simulink model "polaczenie"  (R2013a)
settings: Solver=FixedStepDiscrete  StartTime=0.0  StopTime=inf  FixedStep=0.01  RelTol=1e-3
InitFcn:
  | InitFcn
StopFcn:
  | StopFcn
libraries: aerolibtransform2 x2, aerolibobsolete x2, aerolibconvert2 x2, instrumentlib x2, dspmtrx3 x2
settings Model: Creator=Antonio  LastModifiedBy=Antonio
settings SolverCC: AutoInsertRateTranBlk=on  InsertRTBMode=Always
settings OptimizationCC: LocalBlockOutputs=off  SimCompilerOptimization=On
settings SFSimCC: SFSimEnableDebug=off
settings RTWCC: RTWCompilerOptimization=On

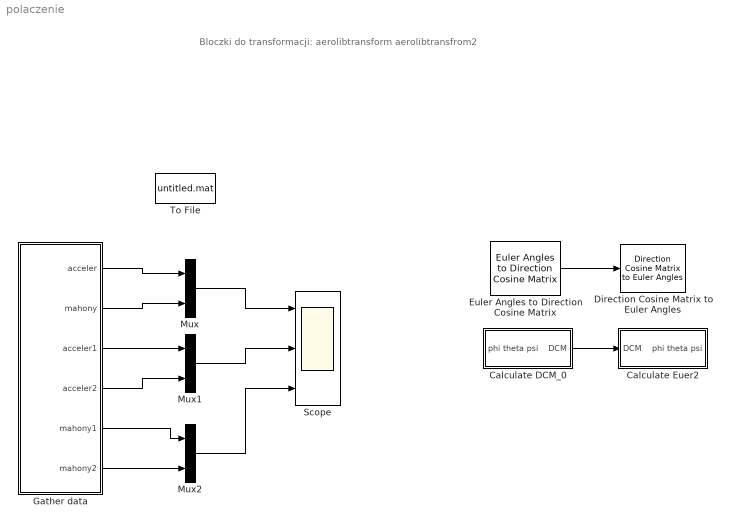
== system polaczenie ==
  note: Bloczki do transformacji:
      | aerolibtransform
      | aerolibtransfrom2
  Calculate DCM_0 : Subsystem
  Calculate Euer2 : Subsystem
  Direction Cosine Matrix to Euler Angles : aerolibobsolete/Direction Cosine Matrix to Euler Angles
  Euler Angles to Direction Cosine Matrix : aerolibobsolete/Euler Angles to  Direction Cosine Matrix
  Gather data : Subsystem
  Mux : Mux  Inputs=2
  Mux1 : Mux  Inputs=2
  Mux2 : Mux  Inputs=2
  Scope : Scope  NumInputPorts=3
      settings: YMin=-200~-175~-175  YMax=200~175~200
  To File : ToFile  SaveFormat=Timeseries
  wires:
  Euler Angles to Direction Cosine Matrix/1 -> Direction Cosine Matrix to Euler Angles/1
  Calculate DCM_0/1(DCM) -> Calculate Euer2/1(DCM)
  Gather data/1(acceler) -> Mux/1
  Gather data/2(mahony) -> Mux/2
  Gather data/3(acceler1) -> Mux1/1
  Gather data/4(acceler2) -> Mux1/2
  Gather data/6(mahony2) -> Mux2/2
  Gather data/5(mahony1) -> Mux2/1
  Mux/1 -> Scope/1
  Mux1/1 -> Scope/2
  Mux2/1 -> Scope/3

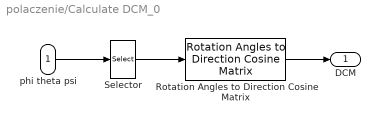
== system polaczenie/Calculate DCM_0 ==
  phi theta psi : Inport
  Rotation Angles to Direction Cosine Matrix : aerolibtransform2/Rotation Angles to Direction Cosine Matrix  rotationOrder=ZYX
  Selector : Selector  InputPortWidth=3  IndexOptions=Index vector (dialog)  Indices=[3 2 1]  OutputSizes=1
  DCM : Outport
  wires:
  Selector/1 -> Rotation Angles to Direction Cosine Matrix/1
  phi theta psi/1 -> Selector/1
  Rotation Angles to Direction Cosine Matrix/1 -> DCM/1

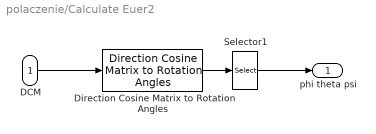
== system polaczenie/Calculate Euer2 ==
  DCM : Inport
  Direction Cosine Matrix to Rotation Angles : aerolibtransform2/Direction Cosine Matrix to Rotation Angles  rotationOrder=ZYX  lim=Default
      settings: AttributesFormatString=Rotation Order: %<rotationOrder>
  Selector1 : Selector  InputPortWidth=3  IndexOptions=Index vector (dialog)  Indices=[3 2 1]  OutputSizes=1
  phi theta psi : Outport
  wires:
  Selector1/1 -> phi theta psi/1
  Direction Cosine Matrix to Rotation Angles/1 -> Selector1/1
  DCM/1 -> Direction Cosine Matrix to Rotation Angles/1

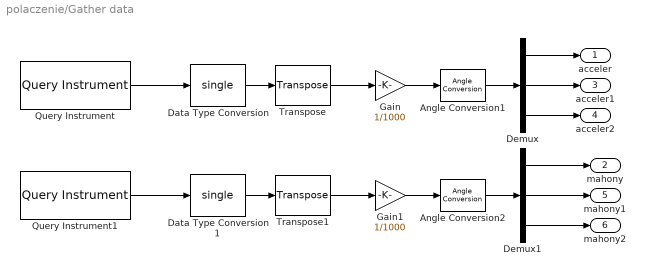
== system polaczenie/Gather data ==
  Angle Conversion1 : aerolibconvert2/Angle Conversion  IU=rad  OU=deg
  Angle Conversion2 : aerolibconvert2/Angle Conversion  IU=rad  OU=deg
  Data Type Conversion : DataTypeConversion  OutDataTypeStr=single  RndMeth=Zero
  Data Type Conversion1 : DataTypeConversion  OutDataTypeStr=single  RndMeth=Zero
  Demux : Demux  Outputs=3
  Demux1 : Demux  Outputs=3
  Gain : Gain  Gain=1/1000
  Gain1 : Gain  Gain=1/1000
  Query Instrument : instrumentlib/Query Instrument  sampleTime=.01  isWorkspaceObject=on  timeout=10  inputBufferSize=512  protocol=Serial  serialPort=COM1  baudRate=9600  gpibVendor=Advantech  boardIndex=0  primaryAddress=1  secondaryAddress=0  visaVendor=Agilent  visaSerialPort=0  chassisIndex=0  logicalAddress=0  tcpRemoteHost='127.0.0.1'  tcpRemotePort=4500  udpRemoteHost='127.0.0.1'  udpRemotePort=9090  visaTCPBoardIndex=0  visaTCPRemoteHost='127.0.0.1'  usbBoardIndex=0  usbManufID=0  usbModelCode=0  usbSerialNumber=0  wsVariableName=board  initAction=None  initCommand='R'  initFunction=get  queryCommand='$R*'  responseFormat=ASCII  asciiFormatting='%d,%d,%d\n'  precision=16-bit unsigned integer  byteOrder=Little endian  valuesToRead=12  removeBytes=off  afterOutputAction=Repeat query for new data  enableFrames=on  frameSize=3
  Query Instrument1 : instrumentlib/Query Instrument  sampleTime=.01  isWorkspaceObject=on  timeout=10  inputBufferSize=512  protocol=Serial  serialPort=COM1  baudRate=9600  gpibVendor=Advantech  boardIndex=0  primaryAddress=1  secondaryAddress=0  visaVendor=Agilent  visaSerialPort=0  chassisIndex=0  logicalAddress=0  tcpRemoteHost='127.0.0.1'  tcpRemotePort=4500  udpRemoteHost='127.0.0.1'  udpRemotePort=9090  visaTCPBoardIndex=0  visaTCPRemoteHost='127.0.0.1'  usbBoardIndex=0  usbManufID=0  usbModelCode=0  usbSerialNumber=0  wsVariableName=board  initAction=None  initCommand='R'  initFunction=get  queryCommand='$M*'  responseFormat=ASCII  asciiFormatting='%d,%d,%d\n'  precision=16-bit unsigned integer  byteOrder=Little endian  valuesToRead=12  removeBytes=off  afterOutputAction=Repeat query for new data  enableFrames=on  frameSize=3
  Transpose : dspmtrx3/Transpose  Hermitian=off  overflowFlag=off
  Transpose1 : dspmtrx3/Transpose  Hermitian=off  overflowFlag=off
  acceler : Outport
  mahony : Outport  Port=2
  acceler1 : Outport  Port=3
  acceler2 : Outport  Port=4
  mahony1 : Outport  Port=5
  mahony2 : Outport  Port=6
  wires:
  Query Instrument/1 -> Data Type Conversion/1
  Data Type Conversion/1 -> Transpose/1
  Transpose/1 -> Gain/1
  Query Instrument1/1 -> Data Type Conversion1/1
  Data Type Conversion1/1 -> Transpose1/1
  Transpose1/1 -> Gain1/1
  Gain/1 -> Angle Conversion1/1
  Gain1/1 -> Angle Conversion2/1
  Demux/1 -> acceler/1
  Demux/2 -> acceler1/1
  Demux/3 -> acceler2/1
  Demux1/1 -> mahony/1
  Demux1/2 -> mahony1/1
  Demux1/3 -> mahony2/1
  Angle Conversion1/1 -> Demux/1
  Angle Conversion2/1 -> Demux1/1
